simulink model "TZ4_SAU_ElPrivod_Nastr_Reg3"  (R2022a)
settings: Solver=ode23tb  StartTime=0.0  StopTime=180  MaxStep=1e-1  RelTol=1e-1
undefined symbols (not defined in the file): CF, DiscIntNeverNeededParam, DT, Es, FI, Filter, PI_reg, RaLa, ReLe, Rsh0, SAU_ElPrivod, SAU_ElPrivod_Nastr_Reg, TagPr, Tokivx, TP, TS, UravDvij, ZU
libraries: spsSeriesRLCBranchLib x18, spsCurrentMeasurementLib x17, spsControlledVoltageSourceLib x8, spsVoltageMeasurementLib x4, dspsigattribs x2, dspstat3 x2, simulink x2, spsIGBTLib x2, spsIdealSwitchLib x1, dspswit3 x1, spsDiodeLib x1, spsDCVoltageSourceLib x1
settings Model: PacingRate=1000  Creator=админ  LastModifiedBy=админ

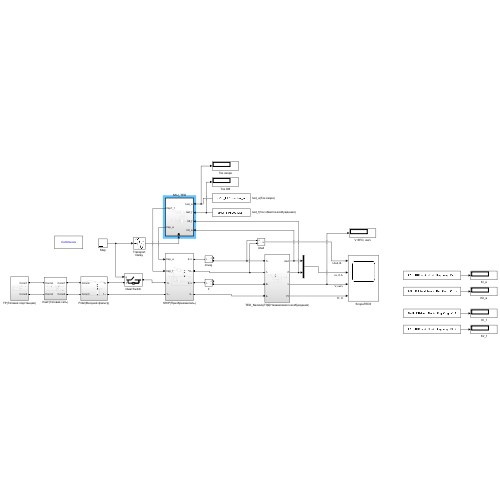
[thumbnail: Simulink's stored preview of the top-level diagram]
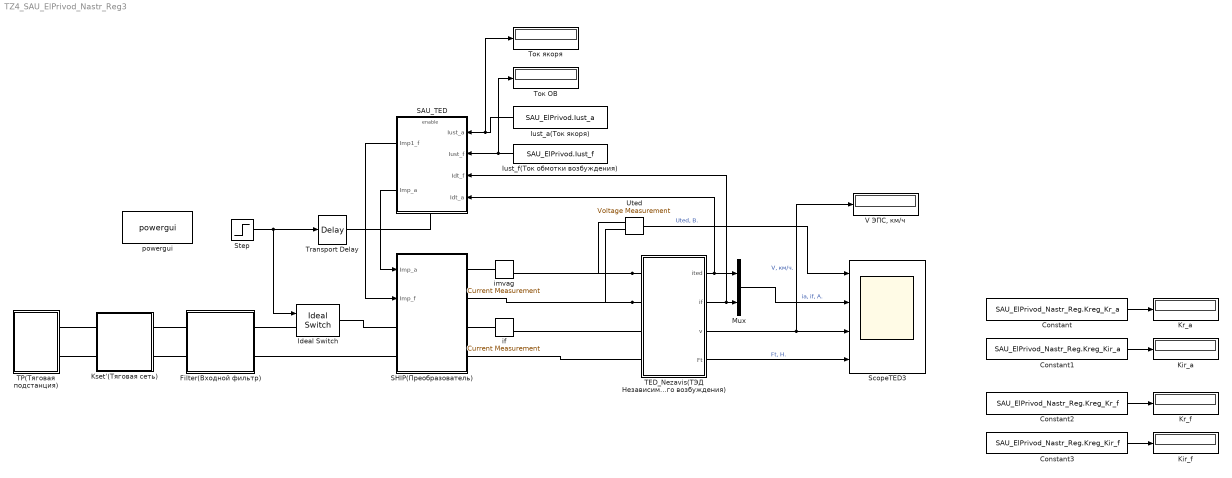
== system TZ4_SAU_ElPrivod_Nastr_Reg3 ==
  Constant : Constant  Value=SAU_ElPrivod_Nastr_Reg.Kreg_Kr_a
  Constant1 : Constant  Value=SAU_ElPrivod_Nastr_Reg.Kreg_Kir_a
  Constant2 : Constant  Value=SAU_ElPrivod_Nastr_Reg.Kreg_Kr_f
  Constant3 : Constant  Value=SAU_ElPrivod_Nastr_Reg.Kreg_Kir_f
  Filter(Входной фильтр) : Subsystem
  Ideal Switch : spsIdealSwitchLib/Ideal Switch  Ron=0.001  Lon=0  IC=0  Rs=1e5  Cs=inf  Measurements=off
  "Iust_a(Ток якоря) " : Constant  Value=SAU_ElPrivod.Iust_a
  Iust_f(Ток обмотки возбуждения) : Constant  Value=SAU_ElPrivod.Iust_f
  Kir_a : Display
  Kir_f : Display
  Kr_a : Display
  Kr_f : Display
  Kset'(Тяговая сеть) : Subsystem
  Mux : Mux  Inputs=2
  SAU_TED : Subsystem
  SHIP(Преобразователь) : Subsystem
  ScopeTED3 : Scope  NumInputPorts=4
  Step : Step  Time=SAU_ElPrivod.Step_time  SampleTime=0
  TED_Nezavis(ТЭД Независимого возбуждения) : Subsystem
  TP(Тяговая подстанция) : Subsystem
  Transport Delay : TransportDelay
  Uted : spsVoltageMeasurementLib/Voltage Measurement  PhasorSimulation=off  OutputType=Complex  PSBequivalent=0
  "V ЭПС, км/ч" : Display
  if : spsCurrentMeasurementLib/Current Measurement  PhasorSimulation=off  OutputType=Complex  PSBequivalent=0
  imvag : spsCurrentMeasurementLib/Current Measurement  PhasorSimulation=off  OutputType=Complex  PSBequivalent=0
  powergui : spspowerguiLib/powergui  Priority=1  SimulationMode=Continuous  SampleTime=50e-6  frequency=60  Iterations=50  frequencyindice=0  Pbase=100e6  ErrMax=1e-4  UnitsV=kV  UnitsW=MW  buscounter=0  FunctionMessages=off  echomessages=off  EnableUseOfTLC=off  CurrentSourceSwitches=off  DisableSnubberDevices=off  DisableRonSwitches=off  DisableVfSwitches=off  DisplayEquations=off  AutomaticDiscreteSolvers=off  SolverType=Tustin/Backward Euler (TBE)  Interpol=off  ExternalGateDelay=off  methode=off  Ts=100  x0status=blocks  SPID=on  SwTol=0  HookPort=off  NonlinearTolerance=1e-4  nMaxIteration=100  ContinueOnMaxIteration=off  RestoreLinks=warning  ResistiveCurrentMeasurement=off  Frange=[0:2:500]  Ylog=off  Xlog=on  ShowGrid=off  save=off  variable=ZData  structure=0  ZoomFFT=off  StartTime=0.0  cycles=1  DisplayStyle=1  fundamental=60  FreqAxis=off  MaxFrequency=1000  frequencyindicesteady=1  RmsSteady=1  display=off
  Ток ОВ : Display
  Ток якоря : Display
  wires:
  TED_Nezavis(ТЭД Независимого возбуждения)/1(ited) -> Mux/1, SAU_TED/4(Idt_a)
  Mux/1 -> ScopeTED3/2  "ia, if, А."
  TED_Nezavis(ТЭД Независимого возбуждения)/3(v) -> "V ЭПС, км/ч"/1, ScopeTED3/3  "V, км/ч."
  Uted/1 -> ScopeTED3/1  "Uted, В."
  TED_Nezavis(ТЭД Независимого возбуждения)/2(if) -> Mux/2, SAU_TED/3(Idt_f)
  TED_Nezavis(ТЭД Независимого возбуждения)/4(Ft) -> ScopeTED3/4  "Ft, Н."
  SAU_TED/2(Imp_a) -> SHIP(Преобразователь)/1(Imp_a)
  SAU_TED/1(Imp1_f) -> SHIP(Преобразователь)/2(Imp_f)
  "Iust_a(Ток якоря) "/1 -> Ток якоря/1, SAU_TED/1(Iust_a)
  Iust_f(Ток обмотки возбуждения)/1 -> Ток ОВ/1, SAU_TED/2(Iust_f)
  Transport Delay/1 -> SAU_TED/Enable
  Step/1 -> Ideal Switch/1, Transport Delay/1
  Constant/1 -> Kr_a/1
  Constant1/1 -> Kir_a/1
  Constant3/1 -> Kir_f/1
  Constant2/1 -> Kr_f/1
  connections:
  TED_Nezavis(ТЭД Независимого возбуждения)/LConn2 -- SHIP(Преобразователь)/RConn2 -- Uted/LConn2
  TED_Nezavis(ТЭД Независимого возбуждения)/LConn1 -- imvag/RConn1 -- Uted/LConn1
  if/LConn1 -- SHIP(Преобразователь)/RConn3
  Kset'(Тяговая сеть)/LConn2 -- TP(Тяговая подстанция)/RConn2
  Kset'(Тяговая сеть)/RConn1 -- Filter(Входной фильтр)/LConn1
  imvag/LConn1 -- SHIP(Преобразователь)/RConn1
  if/RConn1 -- TED_Nezavis(ТЭД Независимого возбуждения)/LConn3
  Kset'(Тяговая сеть)/RConn2 -- Filter(Входной фильтр)/LConn2
  TP(Тяговая подстанция)/RConn1 -- Kset'(Тяговая сеть)/LConn1
  SHIP(Преобразователь)/RConn4 -- TED_Nezavis(ТЭД Независимого возбуждения)/LConn4
  SHIP(Преобразователь)/LConn2 -- Filter(Входной фильтр)/RConn2
  Ideal Switch/RConn1 -- SHIP(Преобразователь)/LConn1
  Ideal Switch/LConn1 -- Filter(Входной фильтр)/RConn1

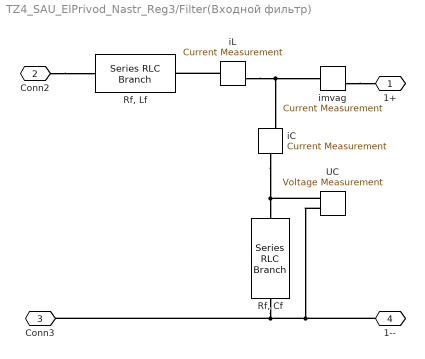
== system TZ4_SAU_ElPrivod_Nastr_Reg3/Filter(Входной фильтр) ==
  "Rf, Cf " : spsSeriesRLCBranchLib/Series RLC Branch  LConnTagsString=__new0  RConnTagsString=__new0  BranchType=RC  Resistance=Filter.R_f  Inductance=1e-3  SetiL0=off  InitialCurrent=0  Capacitance=Filter.C_f  Setx0=off  InitialVoltage=0  Measurements=None
  "Rf, Lf" : spsSeriesRLCBranchLib/Series RLC Branch  LConnTagsString=__new0  RConnTagsString=__new0  BranchType=RL  Resistance=Filter.R_f  Inductance=Filter.L_f  SetiL0=off  InitialCurrent=0  Capacitance=1e-6  Setx0=off  InitialVoltage=0  Measurements=None
  UC : spsVoltageMeasurementLib/Voltage Measurement  PhasorSimulation=off  OutputType=Complex  PSBequivalent=0
  iC : spsCurrentMeasurementLib/Current Measurement  PhasorSimulation=off  OutputType=Complex  PSBequivalent=0
  iL : spsCurrentMeasurementLib/Current Measurement  PhasorSimulation=off  OutputType=Complex  PSBequivalent=0
  imvag : spsCurrentMeasurementLib/Current Measurement  PhasorSimulation=off  OutputType=Complex  PSBequivalent=0
  1+ : PMIOPort  Side=Right
  Conn2 : PMIOPort  Port=2  Side=Left
  Conn3 : PMIOPort  Port=3  Side=Left
  1-- : PMIOPort  Port=4  Side=Right
  connections:
  UC/LConn2 -- 1--/RConn1 -- "Rf, Cf "/RConn1 -- Conn3/RConn1
  iC/LConn1 -- UC/LConn1 -- "Rf, Cf "/LConn1
  iL/RConn1 -- imvag/LConn1 -- iC/RConn1
  iL/LConn1 -- "Rf, Lf"/RConn1
  Conn2/RConn1 -- "Rf, Lf"/LConn1
  imvag/RConn1 -- 1+/RConn1

== system TZ4_SAU_ElPrivod_Nastr_Reg3/Kset'(Тяговая сеть) ==
  "Reks, Leks" : spsSeriesRLCBranchLib/Series RLC Branch  LConnTagsString=__new0  RConnTagsString=__new0  BranchType=RL  Resistance=TS.R_eks  Inductance=TS.L_eks  SetiL0=off  InitialCurrent=0  Capacitance=1e-6  Setx0=off  InitialVoltage=0  Measurements=None
  V1 : spsVoltageMeasurementLib/Voltage Measurement  PhasorSimulation=off  OutputType=Complex  PSBequivalent=0
  i1 : spsCurrentMeasurementLib/Current Measurement  PhasorSimulation=off  OutputType=Complex  PSBequivalent=0
  Conn1 : PMIOPort  Side=Right
  Conn2 : PMIOPort  Port=2  Side=Left
  Conn3 : PMIOPort  Port=3  Side=Left
  Conn4 : PMIOPort  Port=4  Side=Right
  connections:
  "Reks, Leks"/RConn1 -- V1/LConn1 -- i1/LConn1
  Conn2/RConn1 -- "Reks, Leks"/LConn1
  i1/RConn1 -- Conn1/RConn1
  V1/LConn2 -- Conn4/RConn1 -- Conn3/RConn1

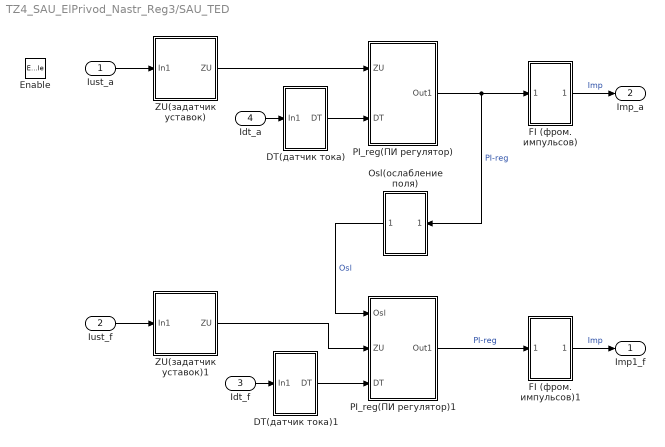
== system TZ4_SAU_ElPrivod_Nastr_Reg3/SAU_TED ==
  Iust_a : Inport
  Iust_f : Inport  Port=2
  Idt_f : Inport  Port=3
  Idt_a : Inport  Port=4
  Enable : EnablePort
  DT(датчик тока) : Subsystem
  DT(датчик тока)1 : Subsystem
  FI (фром. импульсов) : Subsystem
  FI (фром. импульсов)1 : Subsystem
  Osl(ослабление поля) : Subsystem
  PI_reg(ПИ регулятор) : Subsystem
  PI_reg(ПИ регулятор)1 : Subsystem
  ZU(задатчик уставок) : Subsystem
  ZU(задатчик уставок)1 : Subsystem
  Imp1_f : Outport
  Imp_a : Outport  Port=2
  wires:
  PI_reg(ПИ регулятор)/1(Out1) -> Osl(ослабление поля)/1(In1), FI (фром. импульсов)/1(In1)  "PI-reg"
  DT(датчик тока)/1(DT) -> PI_reg(ПИ регулятор)/2(DT)
  ZU(задатчик уставок)/1(ZU) -> PI_reg(ПИ регулятор)/1(ZU)
  FI (фром. импульсов)/1(Out1) -> Imp_a/1  "Imp"
  Idt_a/1 -> DT(датчик тока)/1(In1)
  Iust_a/1 -> ZU(задатчик уставок)/1(In1)
  Iust_f/1 -> ZU(задатчик уставок)1/1(In1)
  Idt_f/1 -> DT(датчик тока)1/1(In1)
  FI (фром. импульсов)1/1(Out1) -> Imp1_f/1  "Imp"
  ZU(задатчик уставок)1/1(ZU) -> PI_reg(ПИ регулятор)1/2(ZU)
  DT(датчик тока)1/1(DT) -> PI_reg(ПИ регулятор)1/3(DT)
  PI_reg(ПИ регулятор)1/1(Out1) -> FI (фром. импульсов)1/1(In1)  "PI-reg"
  Osl(ослабление поля)/1(Osl) -> PI_reg(ПИ регулятор)1/1(Osl)  "Osl"

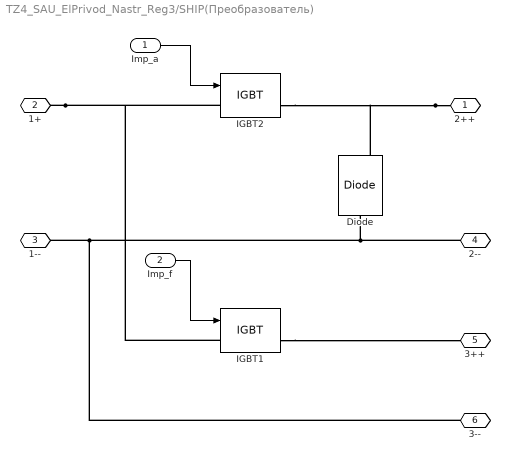
== system TZ4_SAU_ElPrivod_Nastr_Reg3/SHIP(Преобразователь) ==
  Imp_a : Inport
  Imp_f : Inport  Port=2
  Diode : spsDiodeLib/Diode  Ron=Diode.r_t  Lon=0  Vf=0.8  IC=0  UseSnubber=0  Rs=Diode.R_s  Cs=250e-9  Measurements=on
  IGBT1 : spsIGBTLib/IGBT  Ron=IGBT.R_on  Lon=0  Vf=IGBT.V_f  Tf=1e-6  Tt=2e-6  IC=0  Rs=1e5  Cs=inf  Measurements=on
  IGBT2 : spsIGBTLib/IGBT  Ron=IGBT.R_on  Lon=0  Vf=IGBT.V_f  Tf=1e-6  Tt=2e-6  IC=0  Rs=1e5  Cs=inf  Measurements=on
  2++ : PMIOPort  Side=Right
  1+ : PMIOPort  Port=2  Side=Left
  1-- : PMIOPort  Port=3  Side=Left
  2-- : PMIOPort  Port=4  Side=Right
  3++ : PMIOPort  Port=5  Side=Right
  3-- : PMIOPort  Port=6  Side=Right
  wires:
  Imp_a/1 -> IGBT2/1
  Imp_f/1 -> IGBT1/1
  connections:
  1+/RConn1 -- IGBT2/LConn1 -- IGBT1/LConn1
  2++/RConn1 -- IGBT2/RConn1 -- Diode/RConn1
  IGBT1/RConn1 -- 3++/RConn1
  2--/RConn1 -- Diode/LConn1 -- 3--/RConn1 -- 1--/RConn1

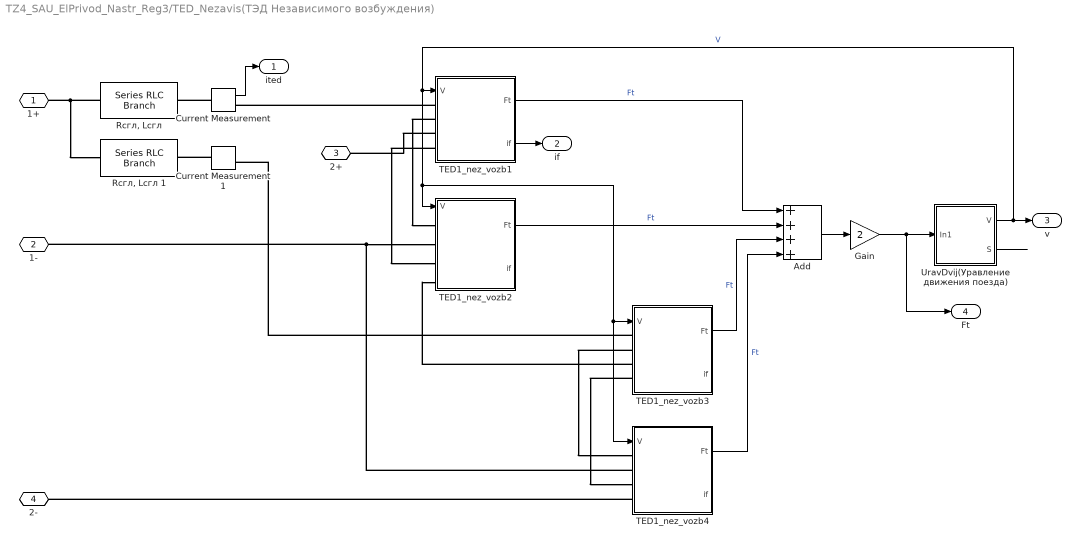
== system TZ4_SAU_ElPrivod_Nastr_Reg3/TED_Nezavis(ТЭД Независимого возбуждения) ==
  Add : Sum  Inputs=++++
  Current Measurement : spsCurrentMeasurementLib/Current Measurement  PhasorSimulation=off  OutputType=Complex  PSBequivalent=0
  Current Measurement1 : spsCurrentMeasurementLib/Current Measurement  PhasorSimulation=off  OutputType=Complex  PSBequivalent=0
  Gain : Gain  Gain=2
  "Rсгл, Lсгл" : spsSeriesRLCBranchLib/Series RLC Branch  LConnTagsString=__new0  RConnTagsString=__new0  BranchType=RL  Resistance=TagPr.R_sgl  Inductance=TagPr.L_sgl  SetiL0=off  InitialCurrent=0  Capacitance=1e-6  Setx0=off  InitialVoltage=0  Measurements=None
  "Rсгл, Lсгл 1" : spsSeriesRLCBranchLib/Series RLC Branch  LConnTagsString=__new0  RConnTagsString=__new0  BranchType=RL  Resistance=TagPr.R_sgl  Inductance=TagPr.L_sgl  SetiL0=off  InitialCurrent=0  Capacitance=1e-6  Setx0=off  InitialVoltage=0  Measurements=None
  TED1_nez_vozb1 : Subsystem
  TED1_nez_vozb2 : Subsystem
  TED1_nez_vozb3 : Subsystem
  TED1_nez_vozb4 : Subsystem
  UravDvij(Уравление движения поезда) : Subsystem
  1+ : PMIOPort  Side=Left
  1- : PMIOPort  Port=2  Side=Left
  2+ : PMIOPort  Port=3  Side=Left
  2- : PMIOPort  Port=4  Side=Left
  ited : Outport
  if : Outport  Port=2
  v : Outport  Port=3
  Ft : Outport  Port=4
  wires:
  TED1_nez_vozb3/1(Ft) -> Add/3  "Ft"
  TED1_nez_vozb1/1(Ft) -> Add/1  "Ft"
  TED1_nez_vozb2/1(Ft) -> Add/2  "Ft"
  Add/1 -> Gain/1
  TED1_nez_vozb4/1(Ft) -> Add/4  "Ft"
  Gain/1 -> Ft/1, UravDvij(Уравление движения поезда)/1(In1)
  Current Measurement/1 -> ited/1
  TED1_nez_vozb1/2(if) -> if/1
  UravDvij(Уравление движения поезда)/2(S) -> ?
  UravDvij(Уравление движения поезда)/1(V) -> v/1, TED1_nez_vozb2/1(V), TED1_nez_vozb3/1(V), TED1_nez_vozb4/1(V), TED1_nez_vozb1/1(V)  "V"
  connections:
  TED1_nez_vozb4/LConn2 -- 1-/RConn1 -- TED1_nez_vozb2/LConn2
  TED1_nez_vozb3/LConn2 -- TED1_nez_vozb4/LConn1
  TED1_nez_vozb1/LConn4 -- TED1_nez_vozb2/LConn3
  TED1_nez_vozb1/LConn2 -- TED1_nez_vozb2/LConn1
  "Rсгл, Lсгл"/LConn1 -- "Rсгл, Lсгл 1"/LConn1 -- 1+/RConn1
  TED1_nez_vozb3/LConn3 -- TED1_nez_vozb2/LConn4
  Current Measurement1/LConn1 -- "Rсгл, Lсгл 1"/RConn1
  Current Measurement/LConn1 -- "Rсгл, Lсгл"/RConn1
  TED1_nez_vozb3/LConn1 -- Current Measurement1/RConn1
  TED1_nez_vozb3/LConn4 -- TED1_nez_vozb4/LConn3
  TED1_nez_vozb1/LConn1 -- Current Measurement/RConn1
  TED1_nez_vozb1/LConn3 -- 2+/RConn1
  TED1_nez_vozb4/LConn4 -- 2-/RConn1

== system TZ4_SAU_ElPrivod_Nastr_Reg3/TP(Тяговая подстанция) ==
  "Rept, Lept" : spsSeriesRLCBranchLib/Series RLC Branch  LConnTagsString=__new0  RConnTagsString=__new0  BranchType=RL  Resistance=TP.R_etp  Inductance=TP.L_etp  SetiL0=off  InitialCurrent=0  Capacitance=1e-6  Setx0=off  InitialVoltage=0  Measurements=None
  Ufid : spsDCVoltageSourceLib/DC Voltage Source  Amplitude=TP.U_tp  Measurements=None
  V2 : spsVoltageMeasurementLib/Voltage Measurement  PhasorSimulation=off  OutputType=Complex  PSBequivalent=0
  i2 : spsCurrentMeasurementLib/Current Measurement  PhasorSimulation=off  OutputType=Complex  PSBequivalent=0
  Conn1 : PMIOPort  Side=Right
  Conn2 : PMIOPort  Port=2  Side=Right
  connections:
  "Rept, Lept"/RConn1 -- V2/LConn1 -- i2/LConn1
  "Rept, Lept"/LConn1 -- Ufid/RConn1
  V2/LConn2 -- Conn2/RConn1 -- Ufid/LConn1
  i2/RConn1 -- Conn1/RConn1

== system TZ4_SAU_ElPrivod_Nastr_Reg3/SAU_TED/DT(датчик тока) ==
  In1 : Inport
  Buffer : Buffer  N=DT.Buffer_size  OutputFrames=off
  Convert 2-D to 1-D : dspsigattribs/Convert 2-D to 1-D
      settings: SourceProductBaseCode=DS
  Filter1 : TransferFcn  Denominator=[DT.T_dt 1]
  Gain : Gain  Gain=DT.K_Gain2
  Mean : dspstat3/Mean  run=off  InputProcessing=Columns as channels (frame based)  reset_popup=None  directionMode=Each column  dimension=1  roiEnable=off  roiType=Rectangles  roiPortion=Entire ROI  roiOutput=Individual statistics for each ROI  roiFlag=off  roundingMode=Floor  overflowMode=off  outputDataTypeStr=Inherit: Same as accumulator  outputMin=[]  outputMax=[]  outputLastDataTypeStr=Inherit: Same as accumulator
  АСР : ZeroOrderHold  SampleTime=DT.T_kv1
  DT : Outport
  wires:
  Filter1/1 -> АСР/1  "Filter"
  АСР/1 -> Buffer/1  "АСР"
  Buffer/1 -> Mean/1
  Gain/1 -> DT/1  "DT"
  Mean/1 -> Convert 2-D to 1-D/1
  In1/1 -> Filter1/1  "Ivx, А"
  Convert 2-D to 1-D/1 -> Gain/1

== system TZ4_SAU_ElPrivod_Nastr_Reg3/SAU_TED/DT(датчик тока)1 ==
  In1 : Inport
  Buffer : Buffer  N=DT.Buffer_size  OutputFrames=off
  Convert 2-D to 1-D : dspsigattribs/Convert 2-D to 1-D
      settings: SourceProductBaseCode=DS
  Filter1 : TransferFcn  Denominator=[DT.T_dt 1]
  Gain : Gain  Gain=DT.K_Gain2
  Mean : dspstat3/Mean  run=off  InputProcessing=Columns as channels (frame based)  reset_popup=None  directionMode=Each column  dimension=1  roiEnable=off  roiType=Rectangles  roiPortion=Entire ROI  roiOutput=Individual statistics for each ROI  roiFlag=off  roundingMode=Floor  overflowMode=off  outputDataTypeStr=Inherit: Same as accumulator  outputMin=[]  outputMax=[]  outputLastDataTypeStr=Inherit: Same as accumulator
  АСР : ZeroOrderHold  SampleTime=DT.T_kv1
  DT : Outport
  wires:
  Convert 2-D to 1-D/1 -> Gain/1
  In1/1 -> Filter1/1  "Ivx, А"
  Mean/1 -> Convert 2-D to 1-D/1
  Gain/1 -> DT/1  "DT"
  Buffer/1 -> Mean/1
  АСР/1 -> Buffer/1  "АСР"
  Filter1/1 -> АСР/1  "Filter"

== system TZ4_SAU_ElPrivod_Nastr_Reg3/SAU_TED/FI (фром. импульсов) ==
  In1 : Inport
  Constant : Constant  Value=FI.frec
  Hit Crossing : HitCross
  Integrator : Integrator  ExternalReset=rising
  Relay : Relay
  Sine Wave : Sin  Frequency=FI.Sine_Wave.freq  SampleTime=0
  Sum : Sum  Inputs=|+-
  Out1 : Outport
  wires:
  Sine Wave/1 -> Hit Crossing/1  "SW"
  Relay/1 -> Out1/1  "Relay"
  In1/1 -> Sum/1  "PI-reg"
  Hit Crossing/1 -> Integrator/2  "HC"
  Integrator/1 -> Sum/2  "Int"
  Constant/1 -> Integrator/1
  Sum/1 -> Relay/1  "Sum"

== system TZ4_SAU_ElPrivod_Nastr_Reg3/SAU_TED/FI (фром. импульсов)1 ==
  In1 : Inport
  Constant : Constant  Value=FI.frec
  Hit Crossing : HitCross
  Integrator : Integrator  ExternalReset=rising
  Relay : Relay
  Sine Wave : Sin  Frequency=FI.Sine_Wave.freq  SampleTime=0
  Sum : Sum  Inputs=|+-
  Out1 : Outport
  wires:
  Sum/1 -> Relay/1  "Sum"
  Constant/1 -> Integrator/1
  Integrator/1 -> Sum/2  "Int"
  Hit Crossing/1 -> Integrator/2  "HC"
  In1/1 -> Sum/1  "PI-reg"
  Relay/1 -> Out1/1  "Relay"
  Sine Wave/1 -> Hit Crossing/1  "SW"

== system TZ4_SAU_ElPrivod_Nastr_Reg3/SAU_TED/Osl(ослабление поля) ==
  In1 : Inport
  Constant : Constant
  Counter : dspswit3/Counter  Direction=Up  CountEvent=Rising edge  CounterSize=User defined  MaxCount=SAU_ElPrivod.Osl.Counter_MaxCount  InitialCount=SAU_ElPrivod.Osl.Counter_InitCount  Output=Count  HitValue=32  ResetInput=off  SamplesPerFrame=1  Ts=1  CntDtype=double  HitDtype=Logical
  Data Type Conversion : DataTypeConversion  SaturateOnIntegerOverflow=off  RndMeth=Floor
  Relational Operator : RelationalOperator  OutDataTypeStr=boolean  RndMeth=Simplest  InputSameDT=off
  Osl : Outport
  wires:
  Counter/1 -> Osl/1  "Counter"
  Relational Operator/1 -> Data Type Conversion/1  "RO"
  Constant/1 -> Relational Operator/2
  In1/1 -> Relational Operator/1  "PI-reg"
  Data Type Conversion/1 -> Counter/1

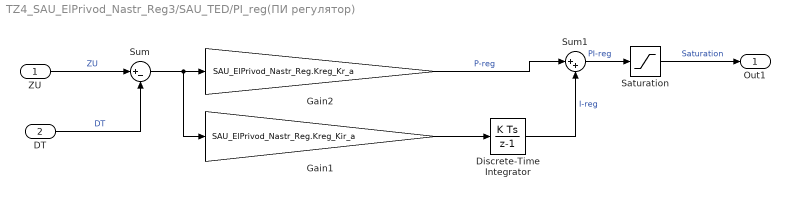
== system TZ4_SAU_ElPrivod_Nastr_Reg3/SAU_TED/PI_reg(ПИ регулятор) ==
  ZU : Inport
  DT : Inport  Port=2
  Discrete-Time Integrator : DiscreteIntegrator  SampleTime=PI_reg.DTI_st  ICPrevOutput=DiscIntNeverNeededParam  ICPrevScaledInput=DiscIntNeverNeededParam
  Gain1 : Gain  Gain=SAU_ElPrivod_Nastr_Reg.Kreg_Kir_a
  Gain2 : Gain  Gain=SAU_ElPrivod_Nastr_Reg.Kreg_Kr_a
  Saturation : Saturate  UpperLimit=PI_reg.StUp_limit  LowerLimit=PI_reg.StLow_limit
  Sum : Sum  Inputs=|+-
  Sum1 : Sum  Inputs=|++
  Out1 : Outport
  wires:
  Sum/1 -> Gain1/1, Gain2/1
  Discrete-Time Integrator/1 -> Sum1/2  "I-reg"
  Gain2/1 -> Sum1/1  "P-reg"
  ZU/1 -> Sum/1  "ZU"
  Gain1/1 -> Discrete-Time Integrator/1
  Saturation/1 -> Out1/1  "Saturation"
  Sum1/1 -> Saturation/1  "PI-reg"
  DT/1 -> Sum/2  "DT"

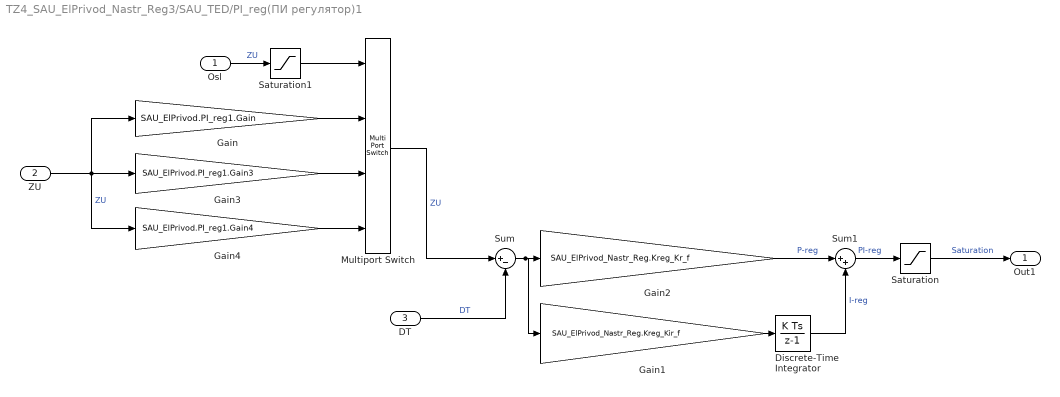
== system TZ4_SAU_ElPrivod_Nastr_Reg3/SAU_TED/PI_reg(ПИ регулятор)1 ==
  Osl : Inport
  ZU : Inport  Port=2
  DT : Inport  Port=3
  Discrete-Time Integrator : DiscreteIntegrator  SampleTime=PI_reg.DTI_st  ICPrevOutput=DiscIntNeverNeededParam  ICPrevScaledInput=DiscIntNeverNeededParam
  Gain : Gain  Gain=SAU_ElPrivod.PI_reg1.Gain
  Gain1 : Gain  Gain=SAU_ElPrivod_Nastr_Reg.Kreg_Kir_f
  Gain2 : Gain  Gain=SAU_ElPrivod_Nastr_Reg.Kreg_Kr_f
  Gain3 : Gain  Gain=SAU_ElPrivod.PI_reg1.Gain3
  Gain4 : Gain  Gain=SAU_ElPrivod.PI_reg1.Gain4
  Multiport Switch : MultiPortSwitch  SaturateOnIntegerOverflow=off  InputSameDT=off
  Saturation : Saturate  UpperLimit=PI_reg.StUp_limit  LowerLimit=PI_reg.StLow_limit
  Saturation1 : Saturate  UpperLimit=SAU_ElPrivod.PI_reg1.StUp_limit  LowerLimit=SAU_ElPrivod.PI_reg1.StLow_limit
  Sum : Sum  Inputs=|+-
  Sum1 : Sum  Inputs=|++
  Out1 : Outport
  wires:
  DT/1 -> Sum/2  "DT"
  Sum1/1 -> Saturation/1  "PI-reg"
  Saturation/1 -> Out1/1  "Saturation"
  Gain1/1 -> Discrete-Time Integrator/1
  ZU/1 -> Gain4/1, Gain3/1, Gain/1  "ZU"
  Gain2/1 -> Sum1/1  "P-reg"
  Discrete-Time Integrator/1 -> Sum1/2  "I-reg"
  Sum/1 -> Gain1/1, Gain2/1
  Osl/1 -> Saturation1/1  "ZU"
  Gain/1 -> Multiport Switch/2
  Gain3/1 -> Multiport Switch/3
  Gain4/1 -> Multiport Switch/4
  Multiport Switch/1 -> Sum/1  "ZU"
  Saturation1/1 -> Multiport Switch/1

== system TZ4_SAU_ElPrivod_Nastr_Reg3/SAU_TED/ZU(задатчик уставок) ==
  In1 : Inport
  Constant : Constant  Value=0
  Discrete-Time Integrator : DiscreteIntegrator  gainval=0.5  SampleTime=1/100  ICPrevOutput=DiscIntNeverNeededParam  ICPrevScaledInput=DiscIntNeverNeededParam
  Gain : Gain  Gain=ZU.K_Gain
  Saturation Dynamic : simulink/Discontinuities/Saturation Dynamic  OutMin=[]  OutMax=[]  OutDataTypeStr=Inherit: Same as second input  OutDataType=fixdt(1, 16)  OutScaling=2^-10  DoSatur=off
  ZU : Outport
  wires:
  Saturation Dynamic/1 -> Gain/1  "SD"
  Discrete-Time Integrator/1 -> Saturation Dynamic/2  "DTI"
  In1/1 -> Saturation Dynamic/1, Discrete-Time Integrator/1  "Ikm"
  Constant/1 -> Saturation Dynamic/3
  Gain/1 -> ZU/1  "Gain"

== system TZ4_SAU_ElPrivod_Nastr_Reg3/SAU_TED/ZU(задатчик уставок)1 ==
  In1 : Inport
  Constant : Constant  Value=0
  Discrete-Time Integrator : DiscreteIntegrator  gainval=1  SampleTime=1/100  ICPrevOutput=DiscIntNeverNeededParam  ICPrevScaledInput=DiscIntNeverNeededParam
  Gain : Gain  Gain=ZU.K_Gain
  Saturation Dynamic : simulink/Discontinuities/Saturation Dynamic  OutMin=[]  OutMax=[]  OutDataTypeStr=Inherit: Same as second input  OutDataType=fixdt(1, 16)  OutScaling=2^-10  DoSatur=off
  ZU : Outport
  wires:
  Gain/1 -> ZU/1  "Gain"
  Constant/1 -> Saturation Dynamic/3
  In1/1 -> Discrete-Time Integrator/1, Saturation Dynamic/1  "Ikm"
  Discrete-Time Integrator/1 -> Saturation Dynamic/2  "DTI"
  Saturation Dynamic/1 -> Gain/1  "SD"

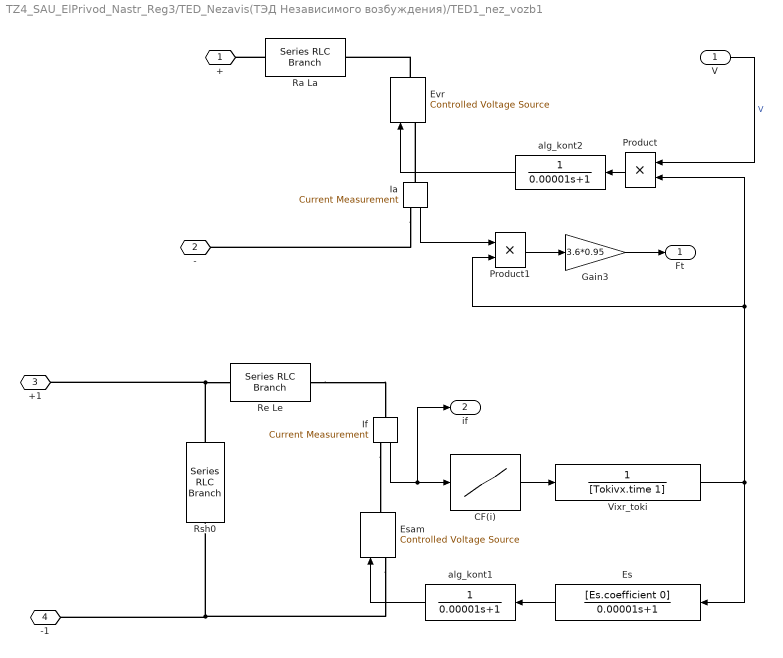
== system TZ4_SAU_ElPrivod_Nastr_Reg3/TED_Nezavis(ТЭД Независимого возбуждения)/TED1_nez_vozb1 ==
  V : Inport
  CF(i) : Lookup_n-D  NumberOfTableDimensions=1  BreakpointsForDimension1=CF.currentvozb  Table=CF.CvF  InternalRulePriority=Speed  RndMeth=Simplest
  Es : TransferFcn  Numerator=[Es.coefficient 0]  Denominator=[0.00001 1]
  Esam : spsControlledVoltageSourceLib/Controlled Voltage Source  Initialize=on  Source_Type=AC  Amplitude=0  Phase=0  Frequency=0  Measurements=None
  Evr : spsControlledVoltageSourceLib/Controlled Voltage Source  Initialize=on  Source_Type=AC  Amplitude=0  Phase=0  Frequency=0  Measurements=None
  Gain3 : Gain  Gain=3.6*0.95
  Ia : spsCurrentMeasurementLib/Current Measurement  PhasorSimulation=off  OutputType=Complex  PSBequivalent=0
  If : spsCurrentMeasurementLib/Current Measurement  PhasorSimulation=off  OutputType=Complex  PSBequivalent=0
  Product : Product
  Product1 : Product
  Ra La : spsSeriesRLCBranchLib/Series RLC Branch  LConnTagsString=__new0  RConnTagsString=__new0  BranchType=RL  Resistance=RaLa.Res  Inductance=RaLa.Ind  SetiL0=off  InitialCurrent=0  Capacitance=1e-6  Setx0=off  InitialVoltage=0  Measurements=None
  Re Le : spsSeriesRLCBranchLib/Series RLC Branch  LConnTagsString=__new0  RConnTagsString=__new0  BranchType=RL  Resistance=ReLe.Res  Inductance=ReLe.Ind  SetiL0=off  InitialCurrent=0  Capacitance=1e-6  Setx0=off  InitialVoltage=0  Measurements=None
  Rsh0 : spsSeriesRLCBranchLib/Series RLC Branch  LConnTagsString=__new0  RConnTagsString=__new0  BranchType=R  Resistance=Rsh0.Res  Inductance=1e-3  SetiL0=off  InitialCurrent=0  Capacitance=1e-6  Setx0=off  InitialVoltage=0  Measurements=None
  Vixr_toki : TransferFcn  Denominator=[Tokivx.time 1]
  alg_kont1 : TransferFcn  Denominator=[0.00001 1]
  alg_kont2 : TransferFcn  Denominator=[0.00001 1]
  + : PMIOPort  Side=Left
  - : PMIOPort  Port=2  Side=Left
  +1 : PMIOPort  Port=3  Side=Left
  -1 : PMIOPort  Port=4  Side=Left
  Ft : Outport
  if : Outport  Port=2
  wires:
  alg_kont2/1 -> Evr/1
  Vixr_toki/1 -> Product1/2, Product/2, Es/1
  Ia/1 -> Product1/1
  Product1/1 -> Gain3/1
  Product/1 -> alg_kont2/1
  Es/1 -> alg_kont1/1
  If/1 -> if/1, CF(i)/1
  alg_kont1/1 -> Esam/1
  CF(i)/1 -> Vixr_toki/1
  V/1 -> Product/1  "V"
  Gain3/1 -> Ft/1
  connections:
  Ia/LConn1 -- Evr/LConn1
  Evr/RConn1 -- Ra La/RConn1
  Rsh0/LConn1 -- +1/RConn1 -- Re Le/LConn1
  If/RConn1 -- Esam/RConn1
  Ia/RConn1 -- -/RConn1
  Esam/LConn1 -- -1/RConn1 -- Rsh0/RConn1
  Re Le/RConn1 -- If/LConn1
  Ra La/LConn1 -- +/RConn1

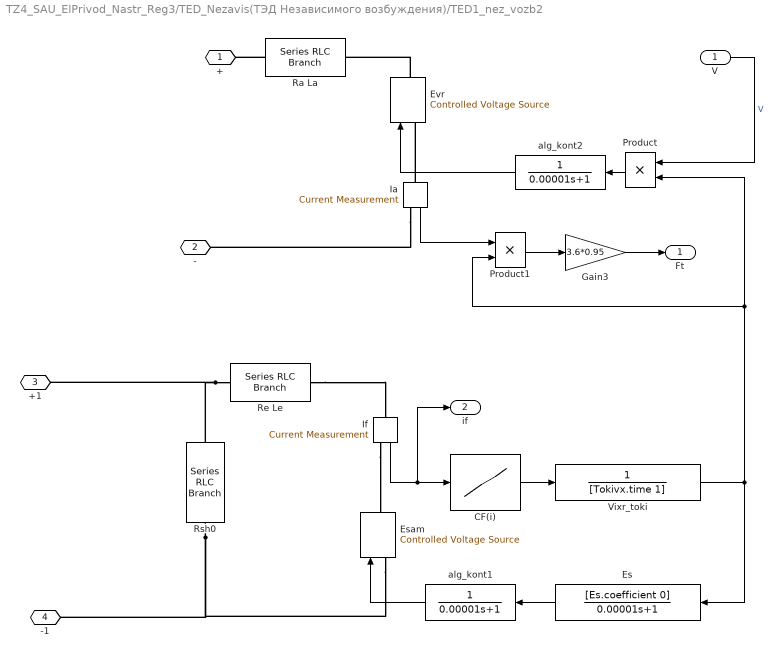
== system TZ4_SAU_ElPrivod_Nastr_Reg3/TED_Nezavis(ТЭД Независимого возбуждения)/TED1_nez_vozb2 ==
  V : Inport
  CF(i) : Lookup_n-D  NumberOfTableDimensions=1  BreakpointsForDimension1=CF.currentvozb  Table=CF.CvF  InternalRulePriority=Speed  RndMeth=Simplest
  Es : TransferFcn  Numerator=[Es.coefficient 0]  Denominator=[0.00001 1]
  Esam : spsControlledVoltageSourceLib/Controlled Voltage Source  Initialize=on  Source_Type=AC  Amplitude=0  Phase=0  Frequency=0  Measurements=None
  Evr : spsControlledVoltageSourceLib/Controlled Voltage Source  Initialize=on  Source_Type=AC  Amplitude=0  Phase=0  Frequency=0  Measurements=None
  Gain3 : Gain  Gain=3.6*0.95
  Ia : spsCurrentMeasurementLib/Current Measurement  PhasorSimulation=off  OutputType=Complex  PSBequivalent=0
  If : spsCurrentMeasurementLib/Current Measurement  PhasorSimulation=off  OutputType=Complex  PSBequivalent=0
  Product : Product
  Product1 : Product
  Ra La : spsSeriesRLCBranchLib/Series RLC Branch  LConnTagsString=__new0  RConnTagsString=__new0  BranchType=RL  Resistance=RaLa.Res  Inductance=RaLa.Ind  SetiL0=off  InitialCurrent=0  Capacitance=1e-6  Setx0=off  InitialVoltage=0  Measurements=None
  Re Le : spsSeriesRLCBranchLib/Series RLC Branch  LConnTagsString=__new0  RConnTagsString=__new0  BranchType=RL  Resistance=ReLe.Res  Inductance=ReLe.Ind  SetiL0=off  InitialCurrent=0  Capacitance=1e-6  Setx0=off  InitialVoltage=0  Measurements=None
  Rsh0 : spsSeriesRLCBranchLib/Series RLC Branch  LConnTagsString=__new0  RConnTagsString=__new0  BranchType=R  Resistance=Rsh0.Res  Inductance=1e-3  SetiL0=off  InitialCurrent=0  Capacitance=1e-6  Setx0=off  InitialVoltage=0  Measurements=None
  Vixr_toki : TransferFcn  Denominator=[Tokivx.time 1]
  alg_kont1 : TransferFcn  Denominator=[0.00001 1]
  alg_kont2 : TransferFcn  Denominator=[0.00001 1]
  + : PMIOPort  Side=Left
  - : PMIOPort  Port=2  Side=Left
  +1 : PMIOPort  Port=3  Side=Left
  -1 : PMIOPort  Port=4  Side=Left
  Ft : Outport
  if : Outport  Port=2
  wires:
  Gain3/1 -> Ft/1
  V/1 -> Product/1  "V"
  CF(i)/1 -> Vixr_toki/1
  alg_kont1/1 -> Esam/1
  If/1 -> CF(i)/1, if/1
  Es/1 -> alg_kont1/1
  Product/1 -> alg_kont2/1
  Product1/1 -> Gain3/1
  Ia/1 -> Product1/1
  Vixr_toki/1 -> Es/1, Product/2, Product1/2
  alg_kont2/1 -> Evr/1
  connections:
  Ra La/LConn1 -- +/RConn1
  Re Le/RConn1 -- If/LConn1
  Rsh0/RConn1 -- -1/RConn1 -- Esam/LConn1
  Ia/RConn1 -- -/RConn1
  If/RConn1 -- Esam/RConn1
  Re Le/LConn1 -- +1/RConn1 -- Rsh0/LConn1
  Evr/RConn1 -- Ra La/RConn1
  Ia/LConn1 -- Evr/LConn1

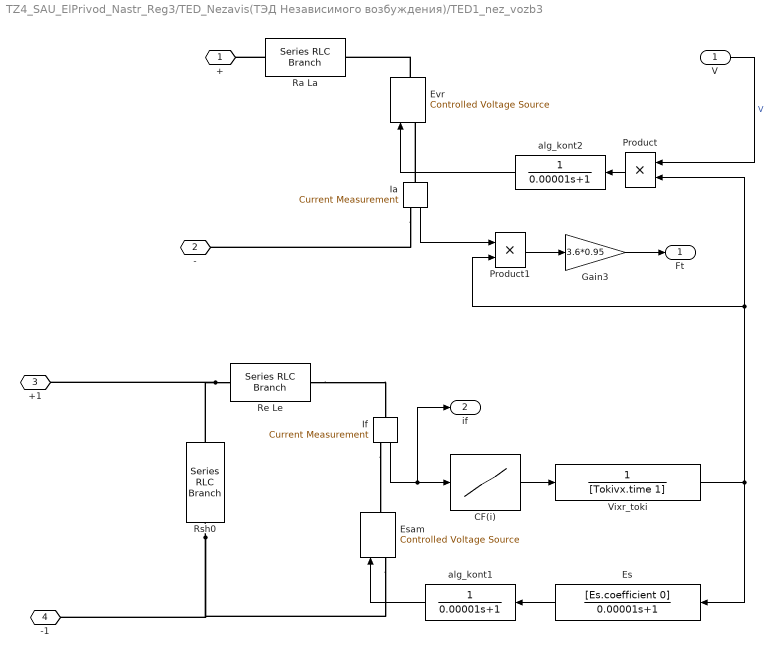
== system TZ4_SAU_ElPrivod_Nastr_Reg3/TED_Nezavis(ТЭД Независимого возбуждения)/TED1_nez_vozb3 ==
  V : Inport
  CF(i) : Lookup_n-D  NumberOfTableDimensions=1  BreakpointsForDimension1=CF.currentvozb  Table=CF.CvF  InternalRulePriority=Speed  RndMeth=Simplest
  Es : TransferFcn  Numerator=[Es.coefficient 0]  Denominator=[0.00001 1]
  Esam : spsControlledVoltageSourceLib/Controlled Voltage Source  Initialize=on  Source_Type=AC  Amplitude=0  Phase=0  Frequency=0  Measurements=None
  Evr : spsControlledVoltageSourceLib/Controlled Voltage Source  Initialize=on  Source_Type=AC  Amplitude=0  Phase=0  Frequency=0  Measurements=None
  Gain3 : Gain  Gain=3.6*0.95
  Ia : spsCurrentMeasurementLib/Current Measurement  PhasorSimulation=off  OutputType=Complex  PSBequivalent=0
  If : spsCurrentMeasurementLib/Current Measurement  PhasorSimulation=off  OutputType=Complex  PSBequivalent=0
  Product : Product
  Product1 : Product
  Ra La : spsSeriesRLCBranchLib/Series RLC Branch  LConnTagsString=__new0  RConnTagsString=__new0  BranchType=RL  Resistance=RaLa.Res  Inductance=RaLa.Ind  SetiL0=off  InitialCurrent=0  Capacitance=1e-6  Setx0=off  InitialVoltage=0  Measurements=None
  Re Le : spsSeriesRLCBranchLib/Series RLC Branch  LConnTagsString=__new0  RConnTagsString=__new0  BranchType=RL  Resistance=ReLe.Res  Inductance=ReLe.Ind  SetiL0=off  InitialCurrent=0  Capacitance=1e-6  Setx0=off  InitialVoltage=0  Measurements=None
  Rsh0 : spsSeriesRLCBranchLib/Series RLC Branch  LConnTagsString=__new0  RConnTagsString=__new0  BranchType=R  Resistance=Rsh0.Res  Inductance=1e-3  SetiL0=off  InitialCurrent=0  Capacitance=1e-6  Setx0=off  InitialVoltage=0  Measurements=None
  Vixr_toki : TransferFcn  Denominator=[Tokivx.time 1]
  alg_kont1 : TransferFcn  Denominator=[0.00001 1]
  alg_kont2 : TransferFcn  Denominator=[0.00001 1]
  + : PMIOPort  Side=Left
  - : PMIOPort  Port=2  Side=Left
  +1 : PMIOPort  Port=3  Side=Left
  -1 : PMIOPort  Port=4  Side=Left
  Ft : Outport
  if : Outport  Port=2
  wires:
  Gain3/1 -> Ft/1
  V/1 -> Product/1  "V"
  CF(i)/1 -> Vixr_toki/1
  alg_kont1/1 -> Esam/1
  If/1 -> CF(i)/1, if/1
  Es/1 -> alg_kont1/1
  Product/1 -> alg_kont2/1
  Product1/1 -> Gain3/1
  Ia/1 -> Product1/1
  Vixr_toki/1 -> Es/1, Product/2, Product1/2
  alg_kont2/1 -> Evr/1
  connections:
  Ra La/LConn1 -- +/RConn1
  Re Le/RConn1 -- If/LConn1
  Rsh0/RConn1 -- -1/RConn1 -- Esam/LConn1
  Ia/RConn1 -- -/RConn1
  If/RConn1 -- Esam/RConn1
  Re Le/LConn1 -- +1/RConn1 -- Rsh0/LConn1
  Evr/RConn1 -- Ra La/RConn1
  Ia/LConn1 -- Evr/LConn1

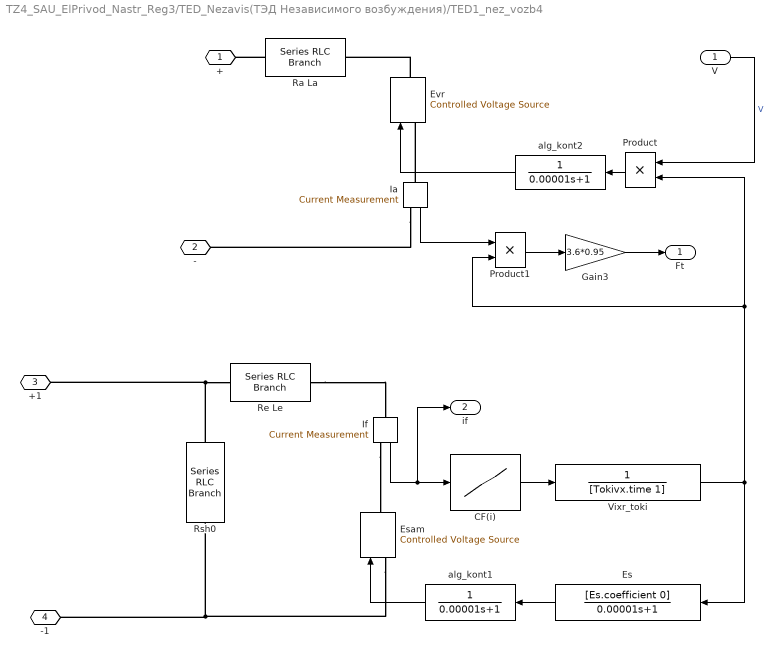
== system TZ4_SAU_ElPrivod_Nastr_Reg3/TED_Nezavis(ТЭД Независимого возбуждения)/TED1_nez_vozb4 ==
  V : Inport
  CF(i) : Lookup_n-D  NumberOfTableDimensions=1  BreakpointsForDimension1=CF.currentvozb  Table=CF.CvF  InternalRulePriority=Speed  RndMeth=Simplest
  Es : TransferFcn  Numerator=[Es.coefficient 0]  Denominator=[0.00001 1]
  Esam : spsControlledVoltageSourceLib/Controlled Voltage Source  Initialize=on  Source_Type=AC  Amplitude=0  Phase=0  Frequency=0  Measurements=None
  Evr : spsControlledVoltageSourceLib/Controlled Voltage Source  Initialize=on  Source_Type=AC  Amplitude=0  Phase=0  Frequency=0  Measurements=None
  Gain3 : Gain  Gain=3.6*0.95
  Ia : spsCurrentMeasurementLib/Current Measurement  PhasorSimulation=off  OutputType=Complex  PSBequivalent=0
  If : spsCurrentMeasurementLib/Current Measurement  PhasorSimulation=off  OutputType=Complex  PSBequivalent=0
  Product : Product
  Product1 : Product
  Ra La : spsSeriesRLCBranchLib/Series RLC Branch  LConnTagsString=__new0  RConnTagsString=__new0  BranchType=RL  Resistance=RaLa.Res  Inductance=RaLa.Ind  SetiL0=off  InitialCurrent=0  Capacitance=1e-6  Setx0=off  InitialVoltage=0  Measurements=None
  Re Le : spsSeriesRLCBranchLib/Series RLC Branch  LConnTagsString=__new0  RConnTagsString=__new0  BranchType=RL  Resistance=ReLe.Res  Inductance=ReLe.Ind  SetiL0=off  InitialCurrent=0  Capacitance=1e-6  Setx0=off  InitialVoltage=0  Measurements=None
  Rsh0 : spsSeriesRLCBranchLib/Series RLC Branch  LConnTagsString=__new0  RConnTagsString=__new0  BranchType=R  Resistance=Rsh0.Res  Inductance=1e-3  SetiL0=off  InitialCurrent=0  Capacitance=1e-6  Setx0=off  InitialVoltage=0  Measurements=None
  Vixr_toki : TransferFcn  Denominator=[Tokivx.time 1]
  alg_kont1 : TransferFcn  Denominator=[0.00001 1]
  alg_kont2 : TransferFcn  Denominator=[0.00001 1]
  + : PMIOPort  Side=Left
  - : PMIOPort  Port=2  Side=Left
  +1 : PMIOPort  Port=3  Side=Left
  -1 : PMIOPort  Port=4  Side=Left
  Ft : Outport
  if : Outport  Port=2
  wires:
  alg_kont2/1 -> Evr/1
  Vixr_toki/1 -> Product1/2, Product/2, Es/1
  Ia/1 -> Product1/1
  Product1/1 -> Gain3/1
  Product/1 -> alg_kont2/1
  Es/1 -> alg_kont1/1
  If/1 -> if/1, CF(i)/1
  alg_kont1/1 -> Esam/1
  CF(i)/1 -> Vixr_toki/1
  V/1 -> Product/1  "V"
  Gain3/1 -> Ft/1
  connections:
  Ia/LConn1 -- Evr/LConn1
  Evr/RConn1 -- Ra La/RConn1
  Rsh0/LConn1 -- +1/RConn1 -- Re Le/LConn1
  If/RConn1 -- Esam/RConn1
  Ia/RConn1 -- -/RConn1
  Esam/LConn1 -- -1/RConn1 -- Rsh0/RConn1
  Re Le/RConn1 -- If/LConn1
  Ra La/LConn1 -- +/RConn1

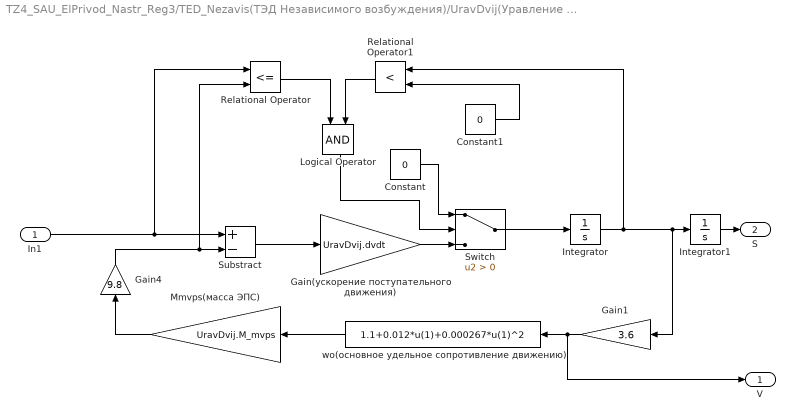
== system TZ4_SAU_ElPrivod_Nastr_Reg3/TED_Nezavis(ТЭД Независимого возбуждения)/UravDvij(Уравление движения поезда) ==
  In1 : Inport
  Constant : Constant  Value=0
  Constant1 : Constant  Value=0
  Gain(ускорение поступательного движения) : Gain  Gain=UravDvij.dvdt
  Gain1 : Gain  Gain=3.6
  Gain4 : Gain  Gain=9.8
  Integrator : Integrator
  Integrator1 : Integrator
  Logical Operator : Logic  AllPortsSameDT=off  OutDataTypeStr=boolean
  Mmvps(масса ЭПС) : Gain  Gain=UravDvij.M_mvps
  Relational Operator : RelationalOperator  Operator=<=  OutDataTypeStr=boolean  RndMeth=Simplest  InputSameDT=off
  Relational Operator1 : RelationalOperator  Operator=<  OutDataTypeStr=boolean  RndMeth=Simplest  InputSameDT=off
  Substract : Sum  Inputs=+-
  Switch : Switch  Criteria=u2 > Threshold  SaturateOnIntegerOverflow=off  InputSameDT=off
  wo(основное удельное сопротивление движению) : Fcn  Expr=1.1+0.012*u(1)+0.000267*u(1)^2
  V : Outport
  S : Outport  Port=2
  wires:
  Switch/1 -> Integrator/1
  wo(основное удельное сопротивление движению)/1 -> Mmvps(масса ЭПС)/1
  Integrator/1 -> Relational Operator1/1, Gain1/1, Integrator1/1
  Gain4/1 -> Relational Operator/2, Substract/2
  Gain1/1 -> V/1, wo(основное удельное сопротивление движению)/1
  In1/1 -> Relational Operator/1, Substract/1
  Constant/1 -> Switch/1
  Relational Operator1/1 -> Logical Operator/2
  Gain(ускорение поступательного движения)/1 -> Switch/3
  Relational Operator/1 -> Logical Operator/1
  Substract/1 -> Gain(ускорение поступательного движения)/1
  Constant1/1 -> Relational Operator1/2
  Logical Operator/1 -> Switch/2
  Integrator1/1 -> S/1
  Mmvps(масса ЭПС)/1 -> Gain4/1
